simulink model "sdruFRSGMRSTx"  (R2014a)
settings: Solver=FixedStepDiscrete  SolverMode=SingleTasking  StartTime=0.0  StopTime=inf  RelTol=1e-3
PreLoadFcn:
  | FRSTxParams = getParamsSdruFRSGMRSTxDemo;
  | frs_Fs = FRSTxParams.SampleRate;
  | frs_toneFreqs = FRSTxParams.ToneFrequencies;
InitFcn:
  | FRSTxParams = getParamsSdruFRSGMRSTxDemo;
  | frs_Fs = FRSTxParams.SampleRate;
  | frs_toneFreqs = FRSTxParams.ToneFrequencies;
undefined symbols (not defined in the file or in its folder): dfilt, mfilt
libraries: dspmlti4 x2, dspsrcs4 x2, dsparch4 x1, sdrublksprivate x1, commsdrhw_v2 x1, dspvision x1
CloseFcn:
  | clear frs_toneFreqs frs_Fs frs_FsFront frs_frameSize FRSTxParams
Description:
  | This model uses Simulink(R) to transmit a Family Radio Service (FRS) signal to Universal Software Radio Peripheral (USRP) hardware.
settings Model: MinMaxOverflowLogging=MinMaxAndOverflow  Creator=The MathWorks Inc.
settings DataIOCC: SignalLoggingSaveFormat=ModelDataLogs  SaveOutput=off  SaveTime=off
settings OptimizationCC: BooleanDataType=off  ExpressionDepthLimit=2147483647  LocalBlockOutputs=off
settings DebuggingCC: AlgebraicLoopMsg=error  UnderspecifiedInitializationDetection=Classic  SingleTaskRateTransMsg=error  ParameterPrecisionLossMsg=none  FcnCallInpInsideContextMsg=UseLocalSettings  StateNameClashWarn=warning
settings HardwareCC: TargetBitPerLong=64  TargetBitPerPointer=64  TargetLongLongMode=on  TargetIntDivRoundTo=Zero  TargetEndianess=LittleEndian  TargetWordSize=64  TargetHWDeviceType=Generic->MATLAB Host Computer  ProdEqTarget=off
settings RTWCC: CustomSourceCode=|
  | #include <stdio.h>
  | #include <stdlib.h>
settings GRTTargetCC: CombineOutputUpdateFcns=off  GRTInterface=on

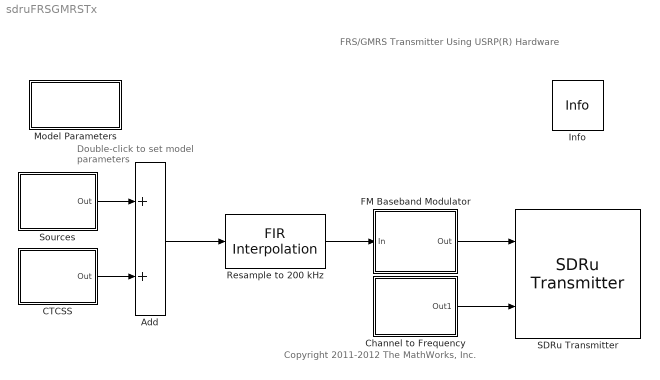
== system sdruFRSGMRSTx ==
  note: FRS/GMRS Transmitter Using USRP(R) Hardware
  note: Copyright 2011-2012 The MathWorks, Inc.
  note: Double-click to
      | set model parameters
  Add : Sum  SampleTime=1/FRSTxParams.SampleRate*FRSTxParams.SourceFrameLength
  CTCSS : Subsystem
      mask Display: disp('CTCSS')
  Channel to Frequency : Subsystem
      mask Display: disp('Channel to\nFrequency');
  FM Baseband Modulator : Subsystem
      mask Display: disp('FM Baseband\nModulator');
  Info : sdrublksprivate/Info  SystemSampleTime=-1
  Model Parameters : Subsystem  mask(Model Parameters){selection=Sound file, tone_freq=880, target_sweep_time=3, channel=12, code=5, amplitude=0.15}
      mask prompts: selection "Signal selection:"; tone_freq "Pure tone frequency (Hz):"; target_sweep_time "Chirp target/sweep time (s):"; channel "Channel (1 to 14):"; code "CTCSS Code (1 to 38):"; amplitude "CTCSS Amplitude:"
      mask help: Specifies model parameters for a simulation run.
      mask init:
      | usrpFRSGMRS_mask(gcbh, 'init', 'trans', selection, tone_freq, ...
      |     target_sweep_time, channel, code, amplitude);
      mask Help: web(usrpdhelp, '-helpbrowser');
      mask TypeOptions selection: Pure tone | Chirp | Sound file
      mask Callback selection: usrpFRSGMRS_mask(gcbh,'cbSignalSelection', 'trans');
      mask Display: disp('Model\nParameters');
  Resample to 200 kHz : dspmlti4/FIR Interpolation  h=FRSTxParams.Numerator  L=FRSTxParams.InterpolationFactor  framing=Enforce single-rate processing  outputBufInitCond=0  InputProcessing=Columns as channels (frame based)  firstCoeffDataTypeStr=Inherit: Same word length as input  firstCoeffLastDataTypeStr=Inherit: Same word length as input  firstCoeffMin=[]  firstCoeffMax=[]  outputDataTypeStr=Inherit: Same as accumulator  outputLastDataTypeStr=Inherit: Same as accumulator  outputMin=[]  outputMax=[]  roundingMode=Floor  overflowMode=off  FilterSource=Specify via dialog  FilterObject=Hm_firinterp
  SDRu Transmitter : commsdrhw_v2/SDRu Transmitter  rxtx=tx  USRP2_IP='192.168.10.2'  centerFrequency=2.45e9  centerFrequencySrc=Input port  loOffset=0  loOffsetSrc=Dialog  gain=FRSTxParams.USRPGain  gainSrc=Dialog  decimInterp=FRSTxParams.USRPInterpolationFactor  decimInterpSrc=Dialog  USRP2_IP_NUM=[49 57 50 46 49 54 56 46 49 48 46 50]  frameLength=362  outputDatatype=int16  overrunUnderrunPort=off  sampleTime=1  dboardInfo=|  HOST_DATA_PORT=30000  HOST_CONTROL_PORT=30001  USRP2_DATA_PORT=32769  USRP2_CONTROL_PORT=32768  bufferMode=Continuous streaming  EnableBurstMode=off  NumFramesInBurst=100
      | dbid: 0
      |           dbName: 'no db found'
      |          freqMin: 0
      |          freqMax: 0
      |          gainMin: 0
      |          gainMax: 0
      |     gainStepSize: 0
  Sources : Subsystem
      mask Display: disp('Sources');
  wires:
  CTCSS/1(Out) -> Add/2
  Add/1 -> Resample to 200 kHz/1
  Channel to Frequency/1(Out1) -> SDRu Transmitter/2
  FM Baseband Modulator/1(Out) -> SDRu Transmitter/1
  Resample to 200 kHz/1 -> FM Baseband Modulator/1(In)
  Sources/1(Out) -> Add/1

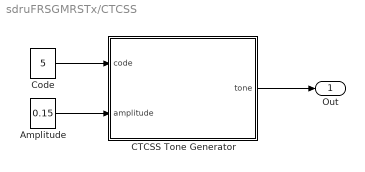
== system sdruFRSGMRSTx/CTCSS ==
  Amplitude : Constant  Value=0.15  VectorParams1D=off  OutDataTypeStr=single  FramePeriod=-1
  CTCSS Tone Generator : MATLAB Function  TreatAsAtomicUnit=on  SystemSampleTime=1/FRSTxParams.SampleRate*FRSTxParams.SourceFrameLength
  Code : Constant  Value=5  VectorParams1D=off  OutDataTypeStr=uint8  FramePeriod=-1
  Out : Outport
  wires:
  Code/1 -> CTCSS Tone Generator/1(code)
  Amplitude/1 -> CTCSS Tone Generator/2(amplitude)
  CTCSS Tone Generator/1(tone) -> Out/1

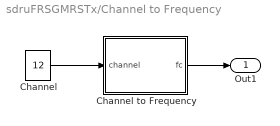
== system sdruFRSGMRSTx/Channel to Frequency ==
  Channel : Constant  Value=12  VectorParams1D=off  OutDataTypeStr=uint8  FramePeriod=-1
  Channel to Frequency : MATLAB Function  TreatAsAtomicUnit=on
  Out1 : Outport
  wires:
  Channel/1 -> Channel to Frequency/1(channel)
  Channel to Frequency/1(fc) -> Out1/1

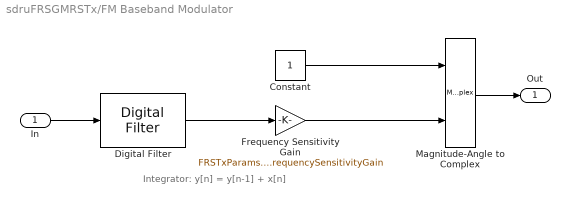
== system sdruFRSGMRSTx/FM Baseband Modulator ==
  note: Integrator:
      | y[n] = y[n-1] + x[n]
  In : Inport
  Constant : Constant  OutDataTypeStr=single  SampleTime=FRSTxParams.AudioInterpolationFactor/FRSTxParams.SampleRate
  Digital Filter : dsparch4/Digital Filter  TypePopup=IIR (poles & zeros)  IIRFiltStruct=Direct form I transposed  AllPoleFiltStruct=Direct form  FIRFiltStruct=Direct form  CoeffSource=Specify via dialog  NumCoeffs=[1]  DenCoeffs=[1 -1]  BiQuadCoeffs=[1 0.3 0.4 1 0.1 0.2]  LatticeCoeffs=[0.2 0.4]  denIgnore=on  FiltPerSampPopup=One filter per frame  IC=0  ICnum=0  ICden=0  roundingMode=Floor  overflowMode=off  ScaleValues=1  scaleValueFracLength=14  stageInFracLength=15  stageOutFracLength=15  FilterSource=Specify via dialog  dfiltObjectName=dfilt.dffir([1 2 1])  InputProcessing=Columns as channels (frame based)
  Frequency Sensitivity Gain : Gain  Gain=FRSTxParams.FrequencySensitivityGain
  Magnitude-Angle to Complex : MagnitudeAngleToComplex
  Out : Outport
  wires:
  Constant/1 -> Magnitude-Angle to Complex/1
  Magnitude-Angle to Complex/1 -> Out/1
  In/1 -> Digital Filter/1
  Digital Filter/1 -> Frequency Sensitivity Gain/1
  Frequency Sensitivity Gain/1 -> Magnitude-Angle to Complex/2

== system sdruFRSGMRSTx/Model Parameters ==
  note: This subsystem is empty.
      | It is used for setting parameter values (in the mask).

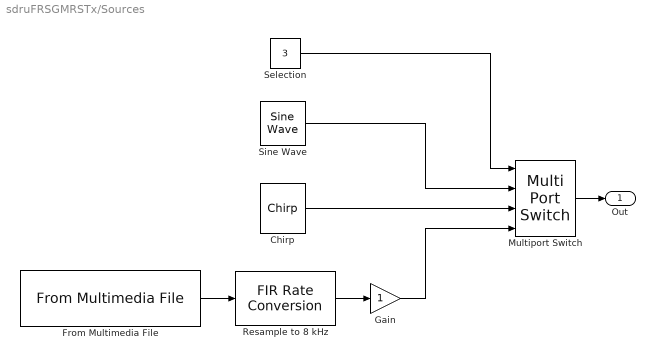
== system sdruFRSGMRSTx/Sources ==
  " Resample to 8 kHz" : dspmlti4/FIR Rate Conversion  L=44  h=[1 1]  M=179  firstCoeffDataTypeStr=Inherit: Same word length as input  firstCoeffLastDataTypeStr=Inherit: Same word length as input  firstCoeffMin=[]  firstCoeffMax=[]  outputDataTypeStr=Inherit: Same as accumulator  outputLastDataTypeStr=Inherit: Same as accumulator  outputMin=[]  outputMax=[]  roundingMode=Floor  overflowMode=off  FilterSource=Filter object  FilterObject=mfilt.firsrc(FRSTxParams.AudioInterpolationFactor,FRSTxParams.AudioDecimationFactor)
  Chirp : dspsrcs4/Chirp  sweep=Linear  mode=Unidirectional  f0=600  f1=1200  t1=3  Tsweep=3  phase=0  Ts=1/FRSTxParams.SampleRate  spf=FRSTxParams.SourceFrameLength  datatype=Single
  From Multimedia File : dspvision/From Multimedia File  inputFilename=speech_dft.avi  loop=on  numPlays=inf  outputStreams=Audio only  videoDataType=single  audioDataType=single  inheritSampleTime=on  userDefinedSampleTime=1/(frs_Fs*(11/4))*33  noAudioOutput=off  isIntensityVideo=off  fourcc=RGB  colorVideoFormat=Separate color signals  outputEOF=off  dataOrg=Column-major  audioFrameSize=FRSTxParams.AudioFrameLength  computeAudioFrameSize=off  outSamplingMode=Frame based
  Gain : Gain
  Multiport Switch : MultiPortSwitch
  Selection : Constant  Value=3
  Sine Wave : dspsrcs4/Sine Wave  Amplitude=1  Frequency=880  Phase=0  SampleMode=Discrete  OutComplex=Real  CompMethod=Trigonometric fcn  TableSize=Speed  SampleTime=1/FRSTxParams.SampleRate  SamplesPerFrame=FRSTxParams.SourceFrameLength  ResetState=Restart at time zero  dataType=single  wordLen=16  udDataType=sfix(16)  fracBitsMode=Best precision  numFracBits=15  OutDataTypeStr=single  LastOutDataTypeStr=single
  Out : Outport
  wires:
  From Multimedia File/1 -> " Resample to 8 kHz"/1
  Sine Wave/1 -> Multiport Switch/2
  " Resample to 8 kHz"/1 -> Gain/1
  Chirp/1 -> Multiport Switch/3
  Selection/1 -> Multiport Switch/1
  Multiport Switch/1 -> Out/1
  Gain/1 -> Multiport Switch/4

== matlab function sdruFRSGMRSTx/CTCSS/CTCSS Tone Generator ==
  data: code input; tone output size=[160 1]; amplitude input; frs_toneFreqs parameter; frs_Fs parameter
function tone  = CTCSS_Gen(code, amplitude, frs_toneFreqs, frs_Fs)
%#codegen

% Generate continuous phase sine wave
%
% PL   Hz     PL   Hz      PL   Hz
% --  ----    --  -----    --  -----
%  1  67.0    12  100.0    32  203.5
%  2  71.9    13  103.5    33  210.7
%  3  74.4    14  107.2    34  218.1
%  4  77.0    15  110.9    35  225.7
%  5  79.7    16  114.8    36  233.6
%  6  82.5    17  118.8    37  241.8
%  7  85.4    18  123.0    38  250.3
%  8  88.5    19  127.3
%  9  91.5    20  131.8
% 10  94.8    21  136.5
% 11  97.4    22  141.3
%             23  146.2
%             24  151.4
%             25  156.7
%             26  162.2
%             27  167.9
%             28  173.8
%             29  179.9
%             30  186.2
%             31  192.8

persistent t0 % The starting time of each frame

Freq      = frs_toneFreqs(code);
frameSize = 160;

if isempty(t0)
    t0 = 0;
end

t = t0 + (0: frameSize-1) / frs_Fs;

t0 = t0 + frameSize/frs_Fs; % The starting time for the next frame

% wrap the time within the first period of the sine wave
if (t0 > 1/Freq)
    t0 = mod(t0, 1/Freq);
end

tone = single(single(amplitude) * sin(2*pi*Freq*t))';

== matlab function sdruFRSGMRSTx/Channel to Frequency/Channel to Frequency ==
  data: channel input uint8; fc output double
function fc = ChanToFreq(channel)
%#codegen
% Map integer channel number to FRS/GMRS center frequencies

fc = convertChan2FreqFRSGMRSDemo(channel);
